simulink model "Modelo_COMPLETO"  (R2023a)
settings: Solver=ode15s  StartTime=0.0  StopTime=100  FixedStep=0.001  MaxStep=0.0003  RelTol=1e-3
model workspace (MAT data in the model file):
  socvcb : containers.Map (value not decoded)
values from neighbouring files (symbols this model uses):
  a_l_max = 0.75    [WorkspaceData.m]
  a_t_max = 0.8    [WorkspaceData.m]
  b_ah = -(b_eqh/i_h - n_h*w_posh*J_eqh/i_h)    [WorkspaceData.m]
  b_at = -double(soluc.b_at)    [WorkspaceData.m]
  b_cx = 1e6    (= 1000000)    [WorkspaceData.m]
  b_cy = 1e7    (= 10000000)    [WorkspaceData.m]
  b_hb = 1.0E+8    (= 100000000)    [WorkspaceData.m]
  b_hd = 8    [WorkspaceData.m]
  b_hEb = 2.2E+9    (= 2200000000)    [WorkspaceData.m]
  b_hm = 18    [WorkspaceData.m]
  b_t = 90    [WorkspaceData.m]
  b_tb = 5e6    (= 5000000)    [WorkspaceData.m]
  b_td = 1.8    [WorkspaceData.m]
  b_tm = 6    [WorkspaceData.m]
  b_tw = 3.0e3    (= 3000)    [WorkspaceData.m]
  b_wu = 1500    [WorkspaceData.m]
  barco_x = 0:0.01:50    [WorkspaceData.m]
  barco_y = interp1(bx_c0,by_c0,barco_x,'previous')    [WorkspaceData.m]
  carro_y = ones(1,20)*45    [WorkspaceData.m]
  constante_frenos = 10    [WorkspaceData.m]
  f = 0.1    [WorkspaceData.m]
  F_D_n_x = ones(1,5)*50    [WorkspaceData.m]
  F_D_n_y = 43:1:47    [WorkspaceData.m]
  F_D_u_x = ones(1,5)*53    [WorkspaceData.m]
  F_D_u_y = 43:1:47    [WorkspaceData.m]
  F_I_n_x = ones(1,5)*-30    [WorkspaceData.m]
  F_I_n_y = 43:1:47    [WorkspaceData.m]
  F_I_u_x = ones(1,5)*-33    [WorkspaceData.m]
  F_I_u_y = 43:1:47    [WorkspaceData.m]
  g = 9.80665    [WorkspaceData.m]
  H_c = 2.5    [WorkspaceData.m]
  i_h = 22    [WorkspaceData.m]
  i_t = 30    [WorkspaceData.m]
  J_hdhEb = 3800    [WorkspaceData.m]
  J_hmhb = 30    [WorkspaceData.m]
  J_td = 1200    [WorkspaceData.m]
  J_tmtb = 7    [WorkspaceData.m]
  K_cy = 1.8e9    (= 1800000000)    [WorkspaceData.m]
  K_sah = -n_h*w_posh^2*J_eqh/i_h    [WorkspaceData.m]
  K_sat = double(soluc.K_sat)    [WorkspaceData.m]
  K_siah = w_posh^3*J_eqh/i_h    [WorkspaceData.m]
  K_siat = -double(soluc.K_siat)    [WorkspaceData.m]
  K_tw = 4.8e5    (= 480000)    [WorkspaceData.m]
  k_wu = 2.36E+9    (= 2360000000)    [WorkspaceData.m]
  M_cmax = 70000    [WorkspaceData.m]
  M_s = 15000    [WorkspaceData.m]
  M_t = 30000    [WorkspaceData.m]
  muelle_x = -35:0.01:0    [WorkspaceData.m]
  muelle_y = interp1(mx_c0,my_c0,muelle_x,'previous')    [WorkspaceData.m]
  pos_i_lh = 45-pos_i_yl    [WorkspaceData.m]
  pos_i_x = -13.5    [WorkspaceData.m]
  pos_i_yl = Y_c0(100*(pos_i_x+30)+1)+1    [WorkspaceData.m]
  r_hd = 0.75    [WorkspaceData.m]
  r_td = 0.5    [WorkspaceData.m]
  riel_x = -35:1:55    [WorkspaceData.m]
  riel_y = ones(1,91)*45    [WorkspaceData.m]
  T_hbMax = 5e4    (= 50000)    [WorkspaceData.m]
  T_hEbMax = 1.1e6    (= 1100000)    [WorkspaceData.m]
  T_s0 = T_s1    (= 0.02)    [WorkspaceData.m]
  T_s1 = 20e-3    (= 0.02)    [WorkspaceData.m]
  T_s2 = 5e-3    (= 0.005)    [WorkspaceData.m]
  T_tbmax = 5e3    (= 5000)    [WorkspaceData.m]
  tau_hm = 1e-3    (= 0.001)    [WorkspaceData.m]
  tau_tm = 1e-3    (= 0.001)    [WorkspaceData.m]
  xx_c0 = -30:0.01:50    [WorkspaceData.m]
  Y_t0 = 45    [WorkspaceData.m]
libraries: simulink x9, vrlib x1
(part 2 of 2)

== stateflow chart Modelo_COMPLETO/Nivel 1 ==
  settings: updateMethod=DISCRETE  sampleTime=T_s1
  state OFF
    state Alimentacion_OFF
    state ON
      note: % Freno desactivado = cerrado/frenando
      state FrenosIzaje [parallel]
        settings: executionOrder=5
        state FrenoIzaje_Act
          entry:
          BRK_h=1;
          detener_izaje=0;
        state FrenoIzaje_Des
          entry:
          BRK_h=0;
          detener_izaje=1;
        (default) -> OFF.ON.FrenosIzaje.FrenoIzaje_Des
        OFF.ON.FrenosIzaje.FrenoIzaje_Act -> OFF.ON.FrenosIzaje.FrenoIzaje_Des : [(abs(w_hm) <=w_hm_min && dl_href_manual==0 && ModoOperac == 1) || Falla_E~=0]
        OFF.ON.FrenosIzaje.FrenoIzaje_Des -> OFF.ON.FrenosIzaje.FrenoIzaje_Act : [(Tmh_disp && (dl_href_manual~=0 || BotonFrenoIzaje==1)||ModoOperac == 0) && Falla_E==0]
      state Activar_TLK [parallel]
        settings: executionOrder=9
        state Verificar
          entry:
          n=500;
        state TLK_desactivado
          entry:
          TLK=0;
          % x_t en metros
          n = ceil((x_td+30)*100/250);
          LOAD = 0;
        state TLK_activado
          entry:
          TLK=1;
          n = ceil((x_td+30)*100/250)*(-1);
          LOAD = 1;
        (default) -> Verificar
        Verificar -> TLK_desactivado [order 2] : [SensoresContacto==1 && ActTLK==0 && ModoOperac==1 && LOAD==1]
        Verificar -> TLK_activado [order 1] : [SensoresContacto==1 && ActTLK==1 && ModoOperac==1 && LOAD==0]
        TLK_desactivado -> Verificar
        TLK_activado -> Verificar
      state ControlBalanceo [parallel]
        settings: executionOrder=11
        state BalanceoON
          entry:
          BC = 1;
        state BalanceoOFF
          entry:
          BC = 0;
        (default) -> BalanceoOFF
        BalanceoON -> BalanceoOFF : [~encenderBalanceo || Falla_E~=0]
        BalanceoOFF -> BalanceoON : [encenderBalanceo]
      state FrenosCarro [parallel]
        settings: executionOrder=6
        state FrenoCarro_Act
          entry:
          BRK_t=1;
          detener_carro=0;
        state FrenoCarro_Des
          entry:
          BRK_t=0;
          detener_carro=1;
        (default) -> FrenoCarro_Des
        FrenoCarro_Act -> FrenoCarro_Des : [(abs(w_tm) <=w_tm_min && dx_tref_manual==0 && ModoOperac == 1) || Falla_E~=0]
        FrenoCarro_Des -> FrenoCarro_Act : [(Tmt_disp && (dx_tref_manual ~= 0 || BotonFrenoCarro==1)||ModoOperac == 0) && Falla_E==0]
      state SenalVida [parallel]
        settings: executionOrder=12
        state EsperandoPulso
          entry:
          HayVida=0;
        state EnvioPulso
          entry:
          HayVida = 1;
        (default) -> EsperandoPulso
        EsperandoPulso -> EnvioPulso : after(500,msec)
        EnvioPulso -> EsperandoPulso : after(20,msec)
      state Frenos_Emergencia_Izaje [parallel]
        settings: executionOrder=2
        state FrenoIzaje_Act
          entry:
          BRK_hE=1;
        state FrenoIzaje_Des
          entry:
          BRK_hE=0;
        (default) -> OFF.ON.Frenos_Emergencia_Izaje.FrenoIzaje_Des
        OFF.ON.Frenos_Emergencia_Izaje.FrenoIzaje_Act -> OFF.ON.Frenos_Emergencia_Izaje.FrenoIzaje_Des : [Control_grua==0]
        OFF.ON.Frenos_Emergencia_Izaje.FrenoIzaje_Des -> OFF.ON.Frenos_Emergencia_Izaje.FrenoIzaje_Act : [Control_grua && Falla_E==0]
      state Sobrevelocidad_Carro_e_Izaje [parallel]
        settings: executionOrder=3
        state espera
        state activo
          state Carro [parallel]
            settings: executionOrder=1
            state Sobrevelocidad_Pos_t
              entry:
              dx_tsv=v_t_max;
            state Verificacion_c
              during:
              dx_tsv=dx_tref_manual;
            state Sobrevelocidad_Neg_t
              entry:
              dx_tsv=-v_t_max;
            (default) -> Verificacion_c
            Verificacion_c -> Sobrevelocidad_Pos_t [order 2] : [dx_tref_manual > v_t_max]
            Sobrevelocidad_Pos_t -> Verificacion_c : [dx_tref_manual <= v_t_max]
            Verificacion_c -> Sobrevelocidad_Neg_t [order 1] : [dx_tref_manual < - v_t_max]
            Sobrevelocidad_Neg_t -> Verificacion_c : [dx_tref_manual >= - v_t_max]
          state Izaje [parallel]
            settings: executionOrder=2
            state Verificacion_I
              during:
              dl_hsv=dl_href_manual;
            state Sobrevelocidad_Pos_t1
              during:
              dl_hsv=v_max_izaje;
            state Sobrevelocidad_Neg_t1
              during:
              dl_hsv=-v_max_izaje;
            (default) -> Verificacion_I
            Verificacion_I -> Sobrevelocidad_Pos_t1 [order 1] : [dl_href_manual > v_max_izaje]
            Sobrevelocidad_Pos_t1 -> Verificacion_I : [dl_href_manual <= v_max_izaje]
            Verificacion_I -> Sobrevelocidad_Neg_t1 [order 2] : [dl_href_manual < - v_max_izaje]
            Sobrevelocidad_Neg_t1 -> Verificacion_I : [dl_href_manual >= - v_max_izaje]
        (default) -> activo
        espera -> activo : [enclave==1]
        activo -> espera : [(TLK==1 &&enclave==0)]
      state DeteccionCableFlojo [parallel]
        settings: executionOrder=1
        state CableTenso
          entry:
          TensionCable = 1;
        state CableFlojo
          entry:
          TensionCable = 0;
        (default) -> CableTenso
        CableTenso -> CableFlojo : [F_hw < TensionMinima]
        CableFlojo -> CableTenso : [F_hw>=TensionMinima]
      state FDC_Carro [parallel]
        settings: executionOrder=8
        state Frenar
          entry:
          ModoOperac=1;
          detener_carro=1;
        state En_Movimiento
          entry:
          detener_carro=0;
        (default) -> OFF.ON.FDC_Carro.En_Movimiento
        OFF.ON.FDC_Carro.Frenar -> OFF.ON.FDC_Carro.En_Movimiento : [(w_tm<=0.3 && w_tm>=0 && dx_tref<0) || (w_tm>=-0.3 && w_tm<=0 && dx_tref>0)]
        OFF.ON.FDC_Carro.En_Movimiento -> OFF.ON.FDC_Carro.Frenar : [(FIN_D_n && dx_tref>0) || (FIN_I_n && dx_tref<0)]
      state Deteccion_de_sobrecarga [parallel]
        entry:
        Sobrecarg=0;
        settings: executionOrder=10
        note: % Si hay sobrecarga se frena el carro y el izaje. Solo se abren los frenos si se desciende manualmente
        state Sobrecarga
          entry:
          Sobrecarg=1;
          BRK_h=0;
          BRK_t=0;
        state CondicionNormal
          entry:
          BRK_h=1;
          BRK_t=1;
        state BajarCarga
          entry:
          BRK_h=1;
          BRK_t=1;
          Sobrecarg=0;
        (default) -> CondicionNormal
        CondicionNormal -> Sobrecarga : [M_cX > M_cmax && TensionCable==1 && Sobrecarg==0 && enclave==1]
        BajarCarga -> Sobrecarga [order 1] : [dl_href_manual < 0]
        BajarCarga -> CondicionNormal [order 2] : [TensionCable==0 ]
        Sobrecarga -> BajarCarga : [dl_href_manual > 0]
      state FDC_Izaje [parallel]
        settings: executionOrder=4
        state Frenar
          entry:
          ModoOperac=1;
          detener_izaje=1;
        state En_Movimiento
          entry:
          detener_izaje=0;
        (default) -> OFF.ON.FDC_Izaje.En_Movimiento
        OFF.ON.FDC_Izaje.Frenar -> OFF.ON.FDC_Izaje.En_Movimiento : [w_hm<=0.3]
        OFF.ON.FDC_Izaje.En_Movimiento -> OFF.ON.FDC_Izaje.Frenar : [(FIN_Sup_n && dl_href<0) || (FIN_Inf_n && dl_href>0)]
      state Cambio_de_modo [parallel]
        settings: executionOrder=7
        state Manual
          entry:
          ModoOperac = 1;
          state Carro [parallel]
            settings: executionOrder=1
            state Activado_carro
              during:
              dx_tref=control_aceleracion_x(dx_tsv);
            state DetenerCarro
              entry:
              dx_tref=0;
            state Proximo_FDC_n_I
              during:
              dx_tref=control_aceleracion_x(dx_tsv*(30+x_td)/11);
            state Proximo_FDC_n_D
              during:
              dx_tref=control_aceleracion_x(dx_tsv*(50-x_td)/11);
            state Sobrecarga_
              entry:
              dx_tref=0;
            (default) -> Activado_carro
            Activado_carro -> Proximo_FDC_n_I [order 4] : [x_td<=-19 && dx_tref_manual<0 && detener_carro==0]
            Activado_carro -> DetenerCarro [order 1] : [detener_carro==1]
            Proximo_FDC_n_I -> Activado_carro : [dx_tref_manual>0 || detener_carro==1]
            DetenerCarro -> Activado_carro : [detener_carro==0]
            Activado_carro -> OFF.ON.Cambio_de_modo.Manual.Carro.Sobrecarga_ [order 2] : [Sobrecarg==1]
            Proximo_FDC_n_D -> Activado_carro : [dx_tref_manual<0|| detener_carro==1]
            OFF.ON.Cambio_de_modo.Manual.Carro.Sobrecarga_ -> Activado_carro : [Sobrecarg==0]
            Activado_carro -> Proximo_FDC_n_D [order 3] : [x_td>=39 && dx_tref_manual>0 && detener_carro==0]
          state Izaje [parallel]
            settings: executionOrder=2
            state Proximo_FDC_n_sup
              during:
              dl_href=control_aceleracion_y(dl_hsv*(l_h-5)/7,0);
            state Activado_izaje
              during:
              dl_href=control_aceleracion_y(dl_hsv,0);
            state DetenerIzaje
              entry:
              dl_href=0;
            state Proximo_FDC_n_Inf
              during:
              dl_href=control_aceleracion_y(dl_hsv*(65-l_h)/10,0);
            state Sobrecarga_
              entry:
              dl_href=0;
              control_aceleracion_y(0,1);
            state Altura_baja
              during:
              dl_href=control_aceleracion_y(dl_href_manual,0)*0.08;
              exit:
              control_aceleracion_y(dl_href,1);
            state TensionCable
              entry:
              dl_href=-2;
            (default) -> Activado_izaje
            DetenerIzaje -> Activado_izaje : [detener_izaje==0]
            Activado_izaje -> Proximo_FDC_n_sup [order 4] : [l_h<=12 && dl_href_manual<0 && detener_izaje==0]
            Activado_izaje -> DetenerIzaje [order 2] : [detener_izaje==1]
            Proximo_FDC_n_sup -> Activado_izaje : [dl_href_manual>0 || detener_izaje==1]
            OFF.ON.Cambio_de_modo.Manual.Izaje.Sobrecarga_ -> Activado_izaje : [Sobrecarg==0]
            Activado_izaje -> Proximo_FDC_n_Inf [order 3] : [l_h>=55 && dl_href_manual>0 && detener_izaje==0]
            Activado_izaje -> OFF.ON.Cambio_de_modo.Manual.Izaje.Sobrecarga_ [order 6] : [Sobrecarg==1]
            Proximo_FDC_n_Inf -> Activado_izaje : [dl_href_manual<0 || detener_izaje==1]
            TensionCable -> Activado_izaje : [TensionCable==1]
            Activado_izaje -> Altura_baja [order 5] : [TLK==1 &&enclave==0]
            Altura_baja -> Activado_izaje : [enclave==1]
            Activado_izaje -> TensionCable [order 1] : [TensionCable==0]
        state Automatico
          entry:
          ModoOperac = 0;
          index = 0;
          x_fin_consigna =destino;    % Este valor tiene que ser aleatorio
          x_inic = x_td;                % Posicion en la que se encuentre
          y_inic= 45-l_h;
          posiciones_ref = generador_consignas(Y_c0_modif,v_max_izaje,x_inic,x_fin_consigna,y_inic,LOAD,T_s1);
          tamano = size(posiciones_ref)
          Kp = 0.2;
          during:
          index = index + 1;
          if (index > tamano(2) && abs(x_tref - x_td)>0.01 && index<index_final)
          dx_tref = Kp*(x_tref - x_td);
          dl_href = 0.3*(l_href - l_h);
          elseif (index <= tamano(2))
          x_tref = posiciones_ref(1,index);
          l_href = posiciones_ref(2,index);
          dx_tref = Kp*(x_tref - x_td);
          dl_href = 0.30*(l_href - l_h);
          else
          index_final = index;
          dx_tref = 0;
          dl_href = 0;
          end
        (default) -> Manual
        Manual -> Automatico : [cambioModo == 1]
        Automatico -> Manual [order 1] : [dx_tref_manual ~= 0 || dl_href_manual ~= 0]
        Automatico -> Manual [order 2] : [FIN_Sup_n || FIN_Inf_n || FIN_D_n || FIN_I_n]
    Alimentacion_OFF -> ON : [Alimentacion==1]
    ON -> Alimentacion_OFF : [Alimentacion==0]
    (default) -> ON
  data: Y_c0_vector_modif function_input; v_max_izaje_valor function_input; x_t_valor function_input; x_fin function_input; y_l_valor function_input; LOADED function_input; consignas function_output; Y_t0 parameter double; a constant double =0; xx_c0 parameter; a_t_max parameter; a_l_max parameter; sample_time function_input; dx_manual function_input; v_maxima_x function_output; dy_manual function_input; v_maxima_y function_output; estado function_input; M_cX input; F_hw input; SensoresContacto input; BC output; HayVida output =1; ModoOperac local; TensionCable local; w_hm input; BRK_h output; BRK_hE output; BRK_t output; w_tm input; Falla_E input; FIN_D_n input; FIN_I_n input; dx_tref_manual input; dx_tref output =0; FIN_Sup_n input; FIN_Inf_n input; dl_href_manual input; dl_href output =0; TLK output =0; M_cmax parameter; v_max_izaje input; BotonFrenoCarro input; BotonFrenoIzaje input; v_t_max local =4; Tmh_disp local =1; Tmt_disp local =1; w_hm_min local =10; w_tm_min local =10; n output =500; LOAD local =0; Sobrecarg local =0; detener_carro local; detener_izaje local; Control_grua input; encenderBalanceo input; ActTLK input; cambioModo input; TensionMinima local =1; Y_c0_modif input; x_fin_consigna local; x_inic local =-14; Alimentacion local =1; l_h input; x_td input; posiciones_ref local size=[2 400000]; enclave input; dl_hsv local =0; dx_tsv local =0; tamano local; T_s1 parameter; Kp local; index_final local =20000; index local; y_inic local; destino input; l_href local =36.5; x_tref local =-14
  function consignas = generador_consignas(Y_c0_vector_modif,v_max_izaje_valor,x_t_valor,x_fin,y_l_valor, LOADED,sample_time):
    | function consignas = generador_consignas(Y_c0_vector_modif,v_max_izaje_valor,x_t_valor,x_fin,y_l_valor, LOADED,sample_time)
    | 
    | 
    | % y_inic = Y_t0-l_valor
    | y_inic = y_l_valor;
    | y_fin = Y_c0_vector_modif(100*(round(x_fin)+30)+1)+2;
    | v_h_max = v_max_izaje_valor;
    | 
    | if(x_fin>x_t_valor)
    |     Y_c0_2 = Y_c0_vector_modif((100*(round(x_t_valor)+30)+1):(100*(round(x_fin)+30)+1));
    |     m = x_t_valor;
    | else
    |     Y_c0_2 = Y_c0_vector_modif((100*(round(x_fin)+30)+1):(100*(round(x_t_valor)+30)+1));
    |     m = x_fin;
    | end
    | 
    | x = ones(1,length(Y_c0_2));
    | for i = 1:length(Y_c0_2)
    |     x(i) = i;
    | end
    | x = (x+m*100)./100;
    | 
    | 
    | 
    | %||=================================================||
    | %||          PTOS PRINCIPALES A SEGUIR              ||
    | %||=================================================||
    | 
    | [B,II] = sort(Y_c0_2,'descend');                % Se ordena de mayor a menor las alturas del perfil de obstaculos           
    | margen_seg = 4;                               % A la altura del perfil se le suma 3.5m de margen de seguridad 
    | 
    | 
    | %------------------FORMA 1---------------------%
    | largo_max = length(find(B>=B(1)));              % Ancho de la parte mas alta del perfil de obstaculos
    | II = II+m*100;
    | 
    | ys_max = [1 1].*B(1)+margen_seg;     
    | if(x_fin>x_t_valor)
    |     xs_max = [II(1), (II(1)+largo_max)]./100;       % Guardo las posiciones x de esas alturas
    |     m=-2;
    | else
    |     xs_max = [(II(1)+largo_max), II(1)]./100; 
    |     m=2;
    | end
    | 
    | %Caso en el que el destino es la parte más alta del perfil de obstáculos
    | if (x_fin>x_t_valor && B(1)==Y_c0_2(length(Y_c0_2))  || x_fin<x_t_valor && B(1)==Y_c0_2(1))
    |     ptos_x = [x_t_valor   x_t_valor   x_t_valor        xs_max(1)       x_fin    x_fin];
    |     ptos_y = [y_inic      y_inic      B(largo_max+1)   ys_max(1)       y_fin    y_fin];
    |     disp('destino alto')
    | 
    | %Caso en el que el inicio es la parte más alta del perfil de obstáculos
    | elseif (x_fin>x_t_valor && B(1)==Y_c0_2(1)  || x_fin<x_t_valor && B(1)==Y_c0_2(length(Y_c0_2)))
    |     ptos_x = [x_t_valor   x_t_valor   x_t_valor     x_fin                x_fin    x_fin];
    |     ptos_y = [y_inic      y_inic      B(1)+2        B(largo_max+1)+3     y_fin    y_fin];
    |     disp('inicio alto')
    | 
    | %Caso en el que la parte más alta se encuentra entre el inicio y el
    | %destino
    | else
    |     ptos_x = [x_t_valor   x_t_valor          xs_max    x_fin+m        x_fin    x_fin];
    |     ptos_y = [y_inic      y_inic                  ys_max    ys_max(2)      y_fin    y_fin];
    |     disp('medio alto')
    | end
    | 
    | 
    | %------------------FORMA 2---------------------%
    | % yn1 = zeros(1, length(Y_c0_2));  
    | % x1 = zeros(1, length(x));  
    | % yn2 = yn1;
    | % x2 = x1;  
    | % k=1;
    | % i=0;
    | % yn1(1)=y_inic;
    | % 
    | % while yn1(k)<B(1)
    | %     i=i+1;
    | %     if Y_c0_2(i)>yn1(k)
    | %         k=k+1;
    | %         yn1(k)=Y_c0_2(i);
    | %         x1(k)=x(i);
    | %     end
    | % end
    | % yn1 = yn1(1:k);
    | % x1 = x1(1:k);
    | % 
    | % i=length(Y_c0_2);
    | % k=1;
    | % yn2(1)=y_fin;
    | % while yn2(k)<B(1)
    | %     i=i-1;
    | %     if Y_c0_2(i)>yn2(k)
    | %         k=k+1;
    | %         yn2(k)=Y_c0_2(i);
    | %         x2(k)=x(i);
    | %     end
    | % end
    | % yn2 = yn2(1:k);
    | % x2 = x2(1:k);
    | % yn2 = flip(yn2);
    | % x2 = flip(x2);
    | % yn3 = [yn1, yn2]+ margen_seg;
    | % x3=[x1, x2];
    | % 
    | % 
    | % ptos_x=ones(1,length(x3)+2);
    | % ptos_y=ones(1,length(yn3)+2);
    | % 
    | % for i=1:length(ptos_x)
    | %     if i<=2
    | %         ptos_x (i)= x_t_valor;
    | %         ptos_y (i)= y_inic;
    | %     elseif i>=(length(ptos_x)-1)
    | %         ptos_x (i)= x_fin;
    | %         ptos_y (i)= y_fin;
    | %     else
    | %         if(x_fin>x_t_valor)
    | %             ptos_x (i)= x3(i-1);
    | %             ptos_y (i)= yn3(i-1);
    | %         else
    | %             ptos_x (i)= x3(length(x3)-i+2);
    | %             ptos_y (i)= yn3(length(x3)-i+2);
    | %         end
    | % 
    | %     end
    | % end
    | %-----------------------------------------------------%
    | 
    | 
    | if LOADED == 1        
    |     ptos_y = ptos_y + 2.5;    % Si hay carga, se modifica el perfil, para que de una consigna de movimiento de la base del spreader
    | end
    | pto_y = ptos_y;
    | ptos_y = 45 - ptos_y;
    | 
    | 
    | 
    | %||=================================================||
    | %||            CÁLCULO DE VELOCIDADES               ||
    | %||=================================================||
    | 
    | % Calculo de tiempos en funcion de las velocidades maximas
    | % v_h_max es un valor de entrada
    | % v_t_max esta en el workspace
    | 
    | delta_x = diff(ptos_x(2:length(ptos_x)));
    | delta_y = diff(ptos_y(2:length(ptos_y)));
    | 
    | t = zeros(1, length(ptos_x));
    | t(1) = 0;
    | t(2) = 0.5;
    | for i = 3:(length(ptos_x)-1)
    |     t_h = abs(delta_y(i-2))/v_h_max;
    |     t_t = abs(delta_x(i-2))/v_t_max;
    |     if t_h > t_t
    |         t(i) = t(i-1) + t_h;
    |     else
    |         t(i) = t(i-1) + t_t;
    |     end
    | end
    | 
    | t(end) = t(end-1) + 1;
    | 
    | % Perfil forzado de traslacion de carro ---- %
    | 
    | tiempo_nuevo = 0:0.5:t(length(t));
    | ptos_xx = interp1(t,ptos_x,tiempo_nuevo,'pchip');    
    | ptos_yy = interp1(t,ptos_y,tiempo_nuevo,'pchip');    
    | 
    | wpts = [ptos_xx; ptos_yy];
    | vellim = 0.9*[-v_t_max v_t_max; -v_h_max v_h_max];
    | accellim = 0.9*[-a_t_max a_t_max; -a_l_max a_l_max];
    | 
    | [q,qd,qdd,tvec] = contopptraj(wpts,vellim,accellim);
    | 
    | tiempo_consig = 0:sample_time:tvec(length(tvec));
    | size(tiempo_consig);
    | consignas = zeros(2,length(tiempo_consig));
    | consignas(1,:) = interp1(tvec,q(1,:),tiempo_consig,'pchip'); 
    | consignas(2,:) = interp1(tvec,q(2,:),tiempo_consig,'pchip'); 
    | 
    | 
    | 
    | %||=================================================||
    | %||                  GRAFICOS                       ||
    | %||=================================================||
    | figure(1)
    | plot(xx_c0,Y_c0_vector_modif);
    | xlim([-30 50])
    | ylim([-20 50])
    | grid on
    | grid minor
    | title('Trayectoria')
    | xlabel('x');
    | ylabel('y');
    | 
    | figure(2)
    | subplot(3,1,1)
    | plot(tvec, q(1,:), 'r')         % Desplazamientos en x
    | hold all
    | plot(tvec, 45-q(2,:), 'b')      % Desplazamientos en y
    | xlabel('t')
    | ylabel('Positions')
    | hold off
    | grid on
    | grid minor
    | 
    | figure(2)
    | subplot(3,1,2)
    | plot(tvec, qd(1,:), 'r')     % Velocidades en x
    | hold all
    | plot(tvec, -qd(2,:), 'b')     % Velocidades en y
    | xlabel('t')
    | ylabel('Velocity')
    | hold off
    | grid on
    | grid minor
    | 
    | figure(2)
    | subplot(3,1,3)
    | plot(tvec, qdd(1,:), 'r')     % Aceleraciones en x
    | hold all
    | plot(tvec, -qdd(2,:), 'b')     % Aceleraciones en y
    | xlabel('t')
    | ylabel('Acceleration')
    | hold off
    | grid on
    | grid minor
    | 
    | figure(1)
    | hold on
    | plot(q(1,:), 45-q(2,:),'r','LineWidth',1);
    | % for i=1:length(ptos_x)
    | %     plot(ptos_x(i),pto_y(i),'b*')
    | % end
    | hold off
    | 
    | 
    | end
  function v_maxima_x = control_aceleracion_x(dx_manual):
    |  function v_maxima_x = control_aceleracion_x(dx_manual)
    | 
    | persistent dx_tref_manual_ant
    | a_max_x=0.8;  %m/s^2
    | dt=0.02;       %20 ms (tiempo de muestreo del statechart)
    | 
    | if isempty(dx_tref_manual_ant)
    |     dx_tref_manual_ant=0;
    | end
    | if abs(dx_manual)>=abs(dx_tref_manual_ant)
    |     if dx_manual>0
    |         v_max=a_max_x*dt+dx_tref_manual_ant;
    |         if dx_manual>v_max
    |              v_maxima_x=v_max;
    |         else 
    |             v_maxima_x=dx_manual;
    |         end
    | 
    |     else 
    |         v_max=-a_max_x*dt+dx_tref_manual_ant;
    |         if dx_manual<v_max
    |             v_maxima_x=v_max;
    |         else 
    |             v_maxima_x=dx_manual;
    |         end
    |     end
    | else
    |     if dx_manual<dx_tref_manual_ant
    |         v_max=-a_max_x*dt+dx_tref_manual_ant;
    |         if dx_manual<v_max
    |              v_maxima_x=v_max;
    |         else 
    |             v_maxima_x=dx_manual;
    |         end
    | 
    |     else 
    |         v_max=a_max_x*dt+dx_tref_manual_ant;
    |         if dx_manual>v_max
    |             v_maxima_x=v_max;
    |         else 
    |             v_maxima_x=dx_manual;
    |         end
    |     end
    | end
    | dx_tref_manual_ant=v_maxima_x;
    | end
  function v_maxima_y = control_aceleracion_y(dy_manual,estado):
    | function v_maxima_y = control_aceleracion_y(dy_manual,estado)
    | 
    | persistent dy_href_manual_ant
    | a_max_y=0.75;  %m/s^2
    | dt=0.02;       %20 ms (tiempo de muestreo del statechart)
    | 
    | if isempty(dy_href_manual_ant)
    |     dy_href_manual_ant=0;
    | end
    | if estado==0
    |     if abs(dy_manual)>=abs(dy_href_manual_ant)
    |         if dy_manual>0
    |             v_max=a_max_y*dt+dy_href_manual_ant;
    |             if dy_manual>v_max
    |                 v_maxima_y=v_max;
    |             else 
    |                 v_maxima_y=dy_manual;
    |             end
    | 
    |         else 
    |             v_max=-a_max_y*dt+dy_href_manual_ant;
    |             if dy_manual<v_max
    |                 v_maxima_y=v_max;
    |             else 
    |                 v_maxima_y=dy_manual;
    |             end
    |         end
    |     else
    |         if dy_manual<dy_href_manual_ant
    |             v_max=-a_max_y*dt+dy_href_manual_ant;
    |             if dy_manual<v_max
    |                  v_maxima_y=v_max;
    |             else 
    |                 v_maxima_y=dy_manual;
    |             end
    | 
    |         else 
    |             v_max=a_max_y*dt+dy_href_manual_ant;
    |             if dy_manual>v_max
    |                 v_maxima_y=v_max;
    |             else 
    |                 v_maxima_y=dy_manual;
    |             end
    |         end
    |     end
    |     dy_href_manual_ant=v_maxima_y;
    | else   
    |     dy_href_manual_ant=dy_manual;
    | end
    | end

== matlab function Modelo_COMPLETO/MATLAB Function ==
  settings: updateMethod=DISCRETE
  data: TLK input; m_l output; F_hw input; dF_hw input; enclave output
function [m_l,enclave] = fcn(TLK, F_hw, dF_hw)
persistent enclavado
persistent masa_promedio
persistent cont
persistent enclavar_masa
persistent masa_enclavada

if isempty(enclavado)
    enclavado=0;
end
if isempty(masa_promedio)
    masa_promedio=zeros(1,200);
end
if isempty(cont)
    cont=0;
end
if isempty(enclavar_masa)
    enclavar_masa=0;
end
if isempty(masa_enclavada)
    masa_enclavada=0;
end

if TLK==1 && enclavar_masa==0
    if dF_hw<10 && F_hw>200000 || enclavado==1
        m_l=F_hw*2/9.81;
        enclave=0;
        enclavado=1;
        cont=cont+1;
        if cont>200
            masa_promedio(1:199)=masa_promedio(2:200);
            masa_promedio(200)=m_l;
            promedio=sum(masa_promedio)/200;
            if promedio<(m_l+1000) && promedio>(m_l-1000)
                enclavar_masa=1;
                masa_enclavada=m_l;
                enclave=1;
            end
            
        else
        masa_promedio(cont)=m_l;
        end
    else
        m_l=60000;
        enclave=0;
    end
      
elseif TLK==0
    enclavado=0;
    enclavar_masa=0;
    cont=0;
    m_l=15000;
    enclave=0;

elseif enclavar_masa==1
    m_l=masa_enclavada;
    enclave=1;
else
    m_l=0;
    enclave=0;
end


end
